simulink model "Strejc_M"  (R2018a)
settings: Solver=VariableStepAuto  StartTime=0.0  StopTime=t  RelTol=1e-3
values from neighbouring files (symbols this model uses):
  k = 18.05    [model.m]
  T0 = 130    [model.m]
  tau = 42.34    [model.m]
  U = 0.95    [model.m]
settings Model: Creator=Kapi  LastModifiedBy=Kapi

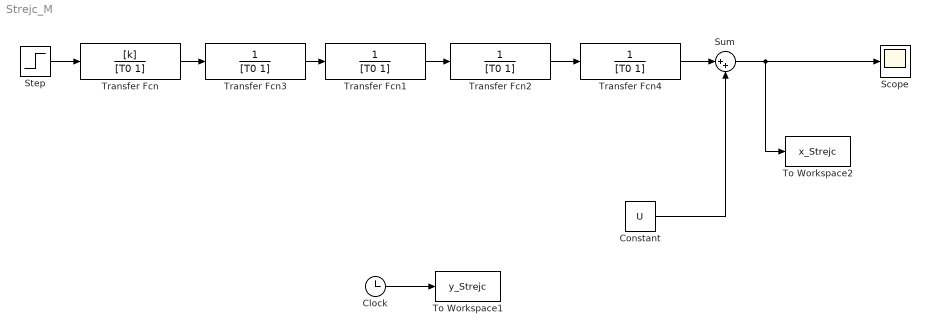
== system Strejc_M ==
  Clock : Clock
  Constant : Constant  Value=U
  Scope : Scope
  Step : Step  Time=tau  SampleTime=0
  Sum : Sum  Inputs=|++
  To Workspace1 : ToWorkspace  VariableName=y_Strejc  SampleTime=-1
  To Workspace2 : ToWorkspace  VariableName=x_Strejc  SampleTime=-1
  Transfer Fcn : TransferFcn  Numerator=[k]  Denominator=[T0 1]
  Transfer Fcn{1..4} (4 alike) : TransferFcn  Denominator=[T0 1]
  wires:
  Step/1 -> Transfer Fcn/1
  Constant/1 -> Sum/2
  Transfer Fcn2/1 -> Transfer Fcn4/1
  Transfer Fcn1/1 -> Transfer Fcn2/1
  Transfer Fcn/1 -> Transfer Fcn3/1
  Transfer Fcn3/1 -> Transfer Fcn1/1
  Clock/1 -> To Workspace1/1
  Sum/1 -> To Workspace2/1, Scope/1
  Transfer Fcn4/1 -> Sum/1
